simulink model "Dynamikk_simulinkmodell"  (R2023b)
settings: Solver=VariableStepAuto  StartTime=0.0  StopTime=500  RelTol=1e-9
values from neighbouring files (symbols this model uses):
  A = [A_x, A_y, A_z, A_phi, A_thetha, A_psi]    [Dynamikk.m]
  Cd = 1.5    [Dynamikk.m]
  F_b = 1    [Dynamikk.m]
  M = M_rb + M_A    [Dynamikk.m]
  r_mb = norm(COB - COM)    [Dynamikk.m]
  rho_vann = 1000    [Dynamikk.m]
  tau = [125;0;0;37.89;0;0]    [Dynamikk.m]
libraries: dspindex x2
settings Model: Creator=anneb  LastModifiedBy=anneb

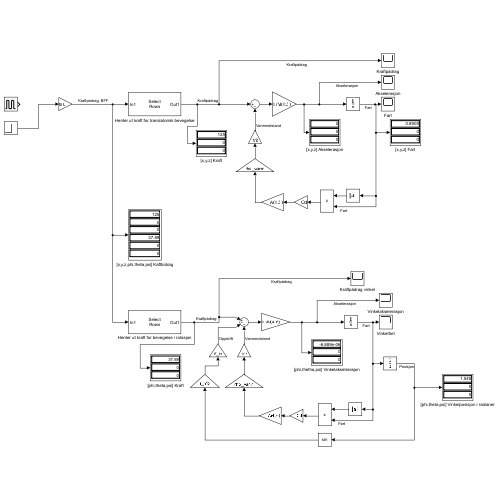
[thumbnail: Simulink's stored preview of the top-level diagram]
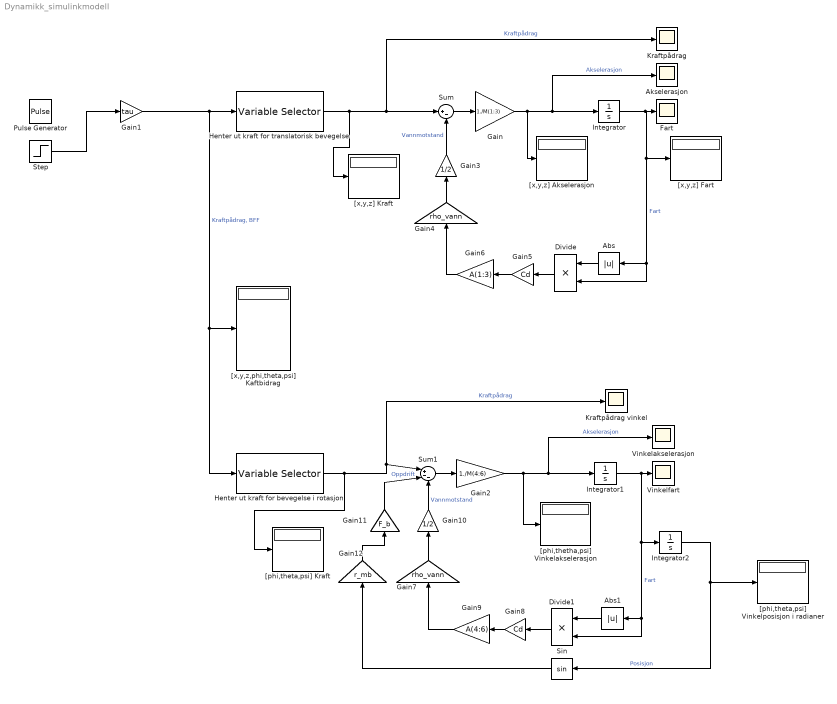
== system Dynamikk_simulinkmodell ==
  Abs : Abs  SaturateOnIntegerOverflow=off
  Abs1 : Abs  SaturateOnIntegerOverflow=off
  Akselerasjon : Scope
  Divide : Product  Inputs=**
  Divide1 : Product  Inputs=**
  Fart : Scope
  Gain : Gain  Gain=1./M(1:3)
  Gain1 : Gain  Gain=tau
  Gain10 : Gain  Gain=1/2
  Gain11 : Gain  Gain=F_b
  Gain12 : Gain  Gain=r_mb
  Gain2 : Gain  Gain=1./M(4:6)
  Gain3 : Gain  Gain=1/2
  Gain4 : Gain  Gain=rho_vann
  Gain5 : Gain  Gain=Cd
  Gain6 : Gain  Gain=A(1:3)
  Gain7 : Gain  Gain=rho_vann
  Gain8 : Gain  Gain=Cd
  Gain9 : Gain  Gain=A(4:6)
  Henter ut kraft for bevegelse i rotasjon : dspindex/Variable Selector  NumInputs=1  rowsOrCols=Rows  IdxMode=Fixed  Elements=[4:6]  ZerOneIdxMode=One-based  errmode=Clip Index  FillMode=off  FillValues=0
  Henter ut kraft for translatorisk bevegelse : dspindex/Variable Selector  NumInputs=1  rowsOrCols=Rows  IdxMode=Fixed  Elements=[1:3]  ZerOneIdxMode=One-based  errmode=Clip Index  FillMode=off  FillValues=0
  Integrator : Integrator
  Integrator1 : Integrator
  Integrator2 : Integrator
  Kraftpådrag : Scope
  Kraftpådrag vinkel : Scope
  Pulse Generator : DiscretePulseGenerator  PulseType=Time based  Period=5  PulseWidth=50
  Sin : Trigonometry
  Step : Step  SampleTime=0
  Sum : Sum  Inputs=|+-
  Sum1 : Sum  Inputs=|+--
  Vinkelakselerasjon : Scope
  Vinkelfart : Scope
  "[phi,theta,psi] Kraft" : Display
  "[phi,theta,psi] Vinkelposisjon i radianer" : Display
  "[phi,thetha,psi] Vinkelakselerasjon" : Display
  "[x,y,z,phi,theta,psi] Kaftbidrag" : Display
  "[x,y,z] Akselerasjon" : Display
  "[x,y,z] Fart" : Display
  "[x,y,z] Kraft" : Display
  wires:
  Henter ut kraft for translatorisk bevegelse/1 -> "[x,y,z] Kraft"/1, Sum/1, Kraftpådrag/1  "Kraftpådrag"
  Gain/1 -> "[x,y,z] Akselerasjon"/1, Akselerasjon/1, Integrator/1  "Akselerasjon"
  Gain1/1 -> "[x,y,z,phi,theta,psi] Kaftbidrag"/1, Henter ut kraft for bevegelse i rotasjon/1, Henter ut kraft for translatorisk bevegelse/1  "Kraftpådrag, BFF"
  Gain2/1 -> "[phi,thetha,psi] Vinkelakselerasjon"/1, Vinkelakselerasjon/1, Integrator1/1  "Akselerasjon"
  Henter ut kraft for bevegelse i rotasjon/1 -> Kraftpådrag vinkel/1, Sum1/1, "[phi,theta,psi] Kraft"/1  "Kraftpådrag"
  Gain6/1 -> Gain4/1
  Divide/1 -> Gain5/1
  Integrator/1 -> Abs/1, Divide/2, "[x,y,z] Fart"/1, Fart/1  "Fart"
  Gain4/1 -> Gain3/1
  Gain5/1 -> Gain6/1
  Abs/1 -> Divide/1
  Sum/1 -> Gain/1
  Gain3/1 -> Sum/2  "Vannmotstand"
  Gain8/1 -> Gain9/1
  Divide1/1 -> Gain8/1
  Gain9/1 -> Gain7/1
  Integrator1/1 -> Vinkelfart/1, Integrator2/1, Abs1/1, Divide1/2  "Fart"
  Abs1/1 -> Divide1/1
  Gain7/1 -> Gain10/1
  Sum1/1 -> Gain2/1
  Gain10/1 -> Sum1/3  "Vannmotstand"
  Integrator2/1 -> "[phi,theta,psi] Vinkelposisjon i radianer"/1, Sin/1  "Posisjon"
  Gain12/1 -> Gain11/1
  Gain11/1 -> Sum1/2  "Oppdrift"
  Sin/1 -> Gain12/1
  Step/1 -> Gain1/1
